simulink model "PMSM_DRIVES_SIMULATION1"  (Simulink 7.8)
settings: Solver=ode23tb  StartTime=0  StopTime=0.1  RelTol=1e-3
libraries: powerlib x6, simulink x2
settings Model: Creator=Nima  LastModifiedBy=Nima  ExtModeTrigMode=oneshot  ExtModeArmWhenConnect=off
settings DataIOCC: LimitDataPoints=off
settings OptimizationCC: BlockReduction=off  BooleanDataType=off  InitFltsAndDblsToZero=on
settings DebuggingCC: SaveWithParameterizedLinksMsg=none  SignalResolutionControl=TryResolveAllWithWarning  SolverPrmCheckMsg=none  MultiTaskDSMMsg=warning  MultiTaskCondExecSysMsg=none  FcnCallInpInsideContextMsg=Use local settings  StrictBusMsg=None
settings HardwareCC: TargetUnknown=on
settings RTWCC: IncludeERTFirstTime=on
settings GRTTargetCC: TargetFcnLib=ansi_tfl_tmw.mat

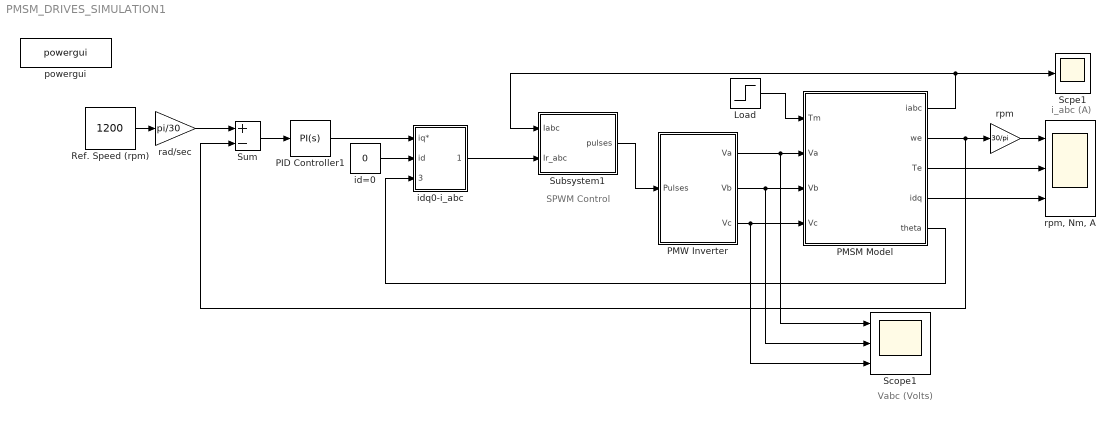
== system PMSM_DRIVES_SIMULATION1 ==
  note: i_abc (A)
  note: SPWM Control
  note: Vabc (Volts)
  " rpm" : Gain  Gain=30/pi  mask{@1=<empty>}
      mask prompts: @1 "Mask Parameter 1:"
      mask StyleString: popup(<empty>)
  Load : Step  Time=0  After=3  SampleTime=0
  PID Controller1 : simulink/Continuous/PID Controller  Controller=PI  TimeDomain=Continuous-time  SampleTime=1  IntegratorMethod=Forward Euler  FilterMethod=Forward Euler  Form=Parallel  P=10  I=2  D=0  N=100  InitialConditionSource=internal  InitialConditionForIntegrator=0  InitialConditionForFilter=0  ExternalReset=none  LimitOutput=off  UpperSaturationLimit=inf  LowerSaturationLimit=-inf  LinearizeAsGain=off  AntiWindupMode=none  Kb=1  TrackingMode=off  Kt=1  PParamMin=[]  PParamMax=[]  IParamMin=[]  IParamMax=[]  DParamMin=[]  DParamMax=[]  NParamMin=[]  NParamMax=[]  KbParamMin=[]  KbParamMax=[]  KtParamMin=[]  KtParamMax=[]  POutMin=[]  POutMax=[]  IOutMin=[]  IOutMax=[]  DOutMin=[]  DOutMax=[]  NOutMin=[]  NOutMax=[]  KbOutMin=[]  KbOutMax=[]  KtOutMin=[]  KtOutMax=[]  IntegratorOutMin=[]  IntegratorOutMax=[]  FilterOutMin=[]  FilterOutMax=[]  SumOutMin=[]  SumOutMax=[]  SumI1OutMin=[]  SumI1OutMax=[]  SumI2OutMin=[]  SumI2OutMax=[]  SumI3OutMin=[]  SumI3OutMax=[]  SumDOutMin=[]  SumDOutMax=[]  SaturationOutMin=[]  SaturationOutMax=[]  IntegratorContinuousStateAttributes=''  IntegratorStateMustResolveToSignalObject=off  IntegratorRTWStateStorageClass=Auto  FilterContinuousStateAttributes=''  FilterStateMustResolveToSignalObject=off  FilterRTWStateStorageClass=Auto
  PMSM Model : Subsystem  mask(PMSM Model ){R=1.4, Ld=0.0066, Lq=0.0058, Yaf=0.1546, J=0.00176, B=0.00038818, P=6}
      mask prompts: R "Stator Resistance R (ohm)"; Ld "Inductance  Ld ( H)"; Lq "Inductance  Lq  ( H)"; Yaf "Rotor Flux constant  Yaf (V/rad/s)"; J "Moment of inertia  J (kgm2)"; B "Friction Vicious gain B (Nm/ rad/s )"; P "Number of Poles P"
      mask help: PMSM drive with constant torque control id=0, at rated speed (60Hz), 30V DC bus voltage..
  PMW Inverter : Subsystem  mask(MOSFET/DIODE 3-Phase Bridge ){Vdc=30}
      mask prompts: Vdc "DC Bus Voltage ( Volts)"
  Ref. Speed (rpm) : Constant  Value=1200
  Scope1 : Scope  NumInputPorts=3
      settings: YMin=-5~-5~-5  YMax=5~5~5
  Scpe1 : Scope
      settings: TimeRange=1  YMin=-10  YMax=10  SaveName=ScopeData6
  Subsystem1 : Subsystem
  Sum : Sum  Inputs=+-  SaturateOnIntegerOverflow=on  InputSameDT=on  OutDataTypeStr=Inherit: Same as first input
  id=0 : Constant  Value=0
  idq0-i_abc : Subsystem  mask(Reference current generator){@1=<empty>}
      mask prompts: @1 "Mask Parameter 1:"
      mask StyleString: popup(<empty>)
  powergui : powerlib/powergui  Priority=2  SimulationMode=Continuous  SolverType=Tustin  SampleTime=0  frequency=60  SPID=off  DisableSnubberDevices=off  DisableRonSwitches=off  DisableVfSwitches=off  SwTol=0  Interpol=off  DisplayEquations=off  FunctionMessages=off  frequencyindice=0  Pbase=100e6  ErrMax=1e-4  Iterations=50  UnitsV=kV  UnitsW=MW  echomessages=off  HookPort=off  EnableUseOfTLC=off  x0status=blocks  RestoreLinks=warning  ResistiveCurrentMeasurement=off  Frange=logspace(0,3,50)  Ylog=off  Xlog=off  ShowGrid=off  save=off  variable=ZData  ZoomFFT=on  StartTime=0.0  cycles=1  DisplayStyle=off  fundamental=60  FreqAxis=off  MaxFrequency=1000  frequencyindicesteady=1  RmsSteady=1  display=off  Ts=0  methode=off
  rad/sec : Gain  Gain=pi/30  mask{@1=<empty>}
      mask prompts: @1 "Mask Parameter 1:"
      mask StyleString: popup(<empty>)
  "rpm, Nm, A" : Scope  NumInputPorts=3
      settings: TimeRange=0.1  YMin=1150~-5~-10  YMax=1240~12.5~10  SaveName=ScopeData3
  wires:
  Sum/1 -> PID Controller1/1
  Ref. Speed (rpm)/1 -> rad/sec/1
  id=0/1 -> idq0-i_abc/2(id)
  Load/1 -> PMSM Model/1(Tm)
  rad/sec/1 -> Sum/1
  PMSM Model/1(iabc) -> Scpe1/1, Subsystem1/1(Iabc)
  PMSM Model/2(we) -> " rpm"/1, Sum/2
  " rpm"/1 -> "rpm, Nm, A"/1
  PMSM Model/3(Te) -> "rpm, Nm, A"/2
  PMW Inverter/1(Va) -> PMSM Model/2(Va), Scope1/1
  PMW Inverter/2(Vb) -> PMSM Model/3(Vb), Scope1/2
  PMW Inverter/3(Vc) -> PMSM Model/4(Vc), Scope1/3
  Subsystem1/1(pulses) -> PMW Inverter/1(Pulses)
  idq0-i_abc/1(irabc) -> Subsystem1/2(Ir_abc)
  PMSM Model/5(theta) -> idq0-i_abc/3(theta)
  PMSM Model/4(idq) -> "rpm, Nm, A"/3
  PID Controller1/1 -> idq0-i_abc/1(iq*)

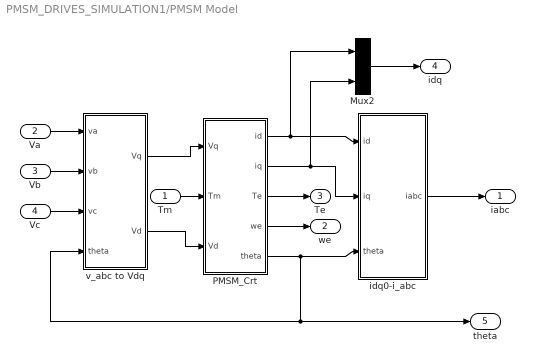
== system PMSM_DRIVES_SIMULATION1/PMSM Model ==
  Tm : Inport
  Va : Inport  Port=2
  Vb : Inport  Port=3
  Vc : Inport  Port=4
  Mux2 : Mux  Inputs=2
  PMSM_Crt : Subsystem  mask{@1=<empty>}
      mask prompts: @1 "Mask Parameter 1:"
      mask StyleString: popup(<empty>)
  idq0-i_abc : Subsystem  mask{@1=<empty>}
      mask prompts: @1 "Mask Parameter 1:"
      mask StyleString: popup(<empty>)
  v_abc to Vdq : Subsystem  mask{@1=<empty>}
      mask prompts: @1 "Mask Parameter 1:"
      mask StyleString: popup(<empty>)
  iabc : Outport
  we : Outport  Port=2
  Te : Outport  Port=3
  idq : Outport  Port=4
  theta : Outport  Port=5
  wires:
  Va/1 -> v_abc to Vdq/1(va)
  Vc/1 -> v_abc to Vdq/3(vc)
  Vb/1 -> v_abc to Vdq/2(vb)
  idq0-i_abc/1(iabc) -> iabc/1
  v_abc to Vdq/1(Vq) -> PMSM_Crt/1(Vq)
  v_abc to Vdq/2(Vd) -> PMSM_Crt/3(Vd)
  PMSM_Crt/1(id) -> idq0-i_abc/1(id), Mux2/1
  PMSM_Crt/2(iq) -> idq0-i_abc/2(iq), Mux2/2
  PMSM_Crt/5(theta) -> theta/1, v_abc to Vdq/4(theta), idq0-i_abc/3(theta)
  PMSM_Crt/4(we) -> we/1
  PMSM_Crt/3(Te) -> Te/1
  Tm/1 -> PMSM_Crt/2(Tm)
  Mux2/1 -> idq/1

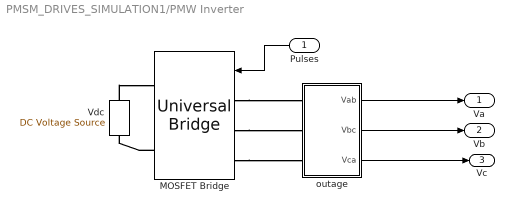
== system PMSM_DRIVES_SIMULATION1/PMW Inverter ==
  Pulses : Inport
  MOSFET Bridge : powerlib/Power Electronics/Universal Bridge  Arms=3  SnubberResistance=1e5  SnubberCapacitance=inf  Device=MOSFET / Diodes  Ron=1e-3  Lon=0  ForwardVoltages="[  0  0  ]"  ForwardVoltage=0  GTOparameters=[ 10e-6 , 20e-6 ]  IGBTparameters=[ 1e-6 , 2e-6 ]  Measurements=None  Measurements_2=None  converterType=Rectifier
  Vdc : powerlib/Electrical Sources/DC Voltage Source  Amplitude=Vdc  Measurements=None
  outage : Subsystem
  Va : Outport
  Vb : Outport  Port=2
  Vc : Outport  Port=3
  wires:
  outage/1(Vab) -> Va/1
  outage/2(Vbc) -> Vb/1
  outage/3(Vca) -> Vc/1
  Pulses/1 -> MOSFET Bridge/1
  connections:
  MOSFET Bridge/LConn1 -- outage/LConn1
  MOSFET Bridge/LConn2 -- outage/LConn2
  MOSFET Bridge/LConn3 -- outage/LConn3
  Vdc/RConn1 -- MOSFET Bridge/RConn1
  MOSFET Bridge/RConn2 -- Vdc/LConn1

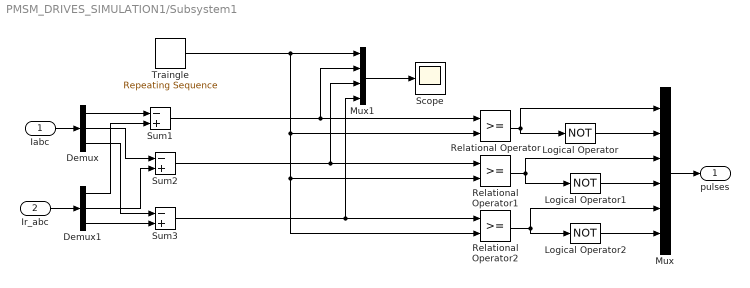
== system PMSM_DRIVES_SIMULATION1/Subsystem1 ==
  Iabc : Inport
  Ir_abc : Inport  Port=2
  Demux : Demux  Outputs=3
  Demux1 : Demux  Outputs=3
  Logical Operator : Logic  Operator=NOT
  Logical Operator1 : Logic  Operator=NOT
  Logical Operator2 : Logic  Operator=NOT
  Mux : Mux  Inputs=6
  Mux1 : Mux
  Relational Operator : RelationalOperator  OutDataTypeStr=boolean
  Relational Operator1 : RelationalOperator  OutDataTypeStr=boolean
  Relational Operator2 : RelationalOperator  OutDataTypeStr=boolean
  Scope : Scope
      settings: YMin=-100  YMax=100  SaveName=ScopeData11
  Sum1 : Sum  Inputs=-+  SaturateOnIntegerOverflow=on  InputSameDT=on  OutDataTypeStr=Inherit: Same as first input
  Sum2 : Sum  Inputs=-+  SaturateOnIntegerOverflow=on  InputSameDT=on  OutDataTypeStr=Inherit: Same as first input
  Sum3 : Sum  Inputs=-+  SaturateOnIntegerOverflow=on  InputSameDT=on  OutDataTypeStr=Inherit: Same as first input
  Traingle : simulink/Sources/Repeating Sequence  rep_seq_t=[0 1/6000/4 3/6000/4 1/6000]  rep_seq_y=[0 -30 30 0]
  pulses : Outport
  wires:
  Iabc/1 -> Demux/1
  Ir_abc/1 -> Demux1/1
  Demux/1 -> Sum1/1
  Demux1/1 -> Sum1/2
  Demux/2 -> Sum2/1
  Demux1/2 -> Sum2/2
  Demux/3 -> Sum3/1
  Demux1/3 -> Sum3/2
  Relational Operator/1 -> Logical Operator/1, Mux/1
  Logical Operator/1 -> Mux/2
  Relational Operator1/1 -> Mux/3, Logical Operator1/1
  Logical Operator1/1 -> Mux/4
  Relational Operator2/1 -> Logical Operator2/1, Mux/5
  Logical Operator2/1 -> Mux/6
  Mux/1 -> pulses/1
  Sum1/1 -> Relational Operator/1, Mux1/2
  Sum2/1 -> Relational Operator1/1, Mux1/3
  Sum3/1 -> Relational Operator2/1, Mux1/4
  Traingle/1 -> Relational Operator2/2, Relational Operator1/2, Relational Operator/2, Mux1/1
  Mux1/1 -> Scope/1

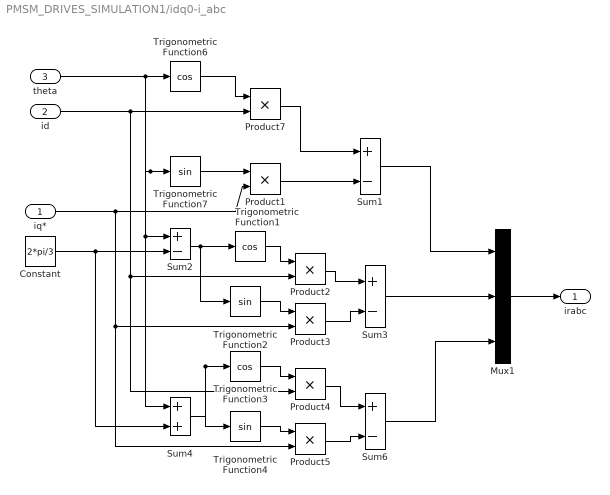
== system PMSM_DRIVES_SIMULATION1/idq0-i_abc ==
  iq* : Inport
  id : Inport  Port=2
  theta : Inport  Port=3
  Constant : Constant  Value=2*pi/3
  Mux1 : Mux  Inputs=3
  Product{1..5,7} (6 alike) : Product  SaturateOnIntegerOverflow=on  RndMeth=Zero  InputSameDT=on  OutDataTypeStr=Inherit: Same as first input
  Sum{1..3,6} (4 alike) : Sum  Inputs=+-  SaturateOnIntegerOverflow=on  InputSameDT=on  OutDataTypeStr=Inherit: Same as first input
  Sum4 : Sum  SaturateOnIntegerOverflow=on  InputSameDT=on  OutDataTypeStr=Inherit: Same as first input
  Trigonometric Function1 : Trigonometry  Operator=cos
  Trigonometric Function2 : Trigonometry
  Trigonometric Function3 : Trigonometry  Operator=cos
  Trigonometric Function4 : Trigonometry
  Trigonometric Function6 : Trigonometry  Operator=cos
  Trigonometric Function7 : Trigonometry
  irabc : Outport
  wires:
  theta/1 -> Trigonometric Function6/1, Trigonometric Function7/1, Sum2/1, Sum4/1
  Trigonometric Function6/1 -> Product7/1
  Trigonometric Function7/1 -> Product1/1
  id/1 -> Product7/2, Product2/2, Product4/2
  Product1/1 -> Sum1/2
  Product7/1 -> Sum1/1
  Sum2/1 -> Trigonometric Function1/1, Trigonometric Function2/1
  Trigonometric Function1/1 -> Product2/1
  Trigonometric Function2/1 -> Product3/1
  Product3/1 -> Sum3/2
  Product2/1 -> Sum3/1
  Sum3/1 -> Mux1/2
  Sum4/1 -> Trigonometric Function3/1, Trigonometric Function4/1
  Trigonometric Function3/1 -> Product4/1
  Trigonometric Function4/1 -> Product5/1
  Product4/1 -> Sum6/1
  Product5/1 -> Sum6/2
  Sum6/1 -> Mux1/3
  Mux1/1 -> irabc/1
  iq*/1 -> Product1/2, Product3/2, Product5/2
  Constant/1 -> Sum2/2, Sum4/2
  Sum1/1 -> Mux1/1

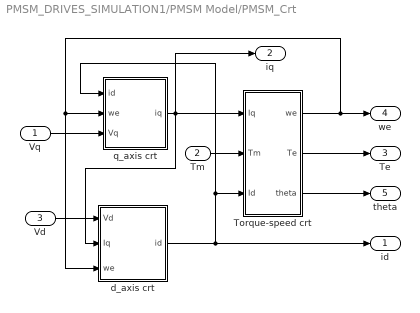
== system PMSM_DRIVES_SIMULATION1/PMSM Model/PMSM_Crt ==
  Vq : Inport
  Tm : Inport  Port=2
  Vd : Inport  Port=3
  Torque-speed crt : Subsystem  mask{@1=<empty>}
      mask prompts: @1 "Mask Parameter 1:"
      mask StyleString: popup(<empty>)
  d_axis crt : Subsystem  mask{@1=<empty>}
      mask prompts: @1 "Mask Parameter 1:"
      mask StyleString: popup(<empty>)
  q_axis crt : Subsystem  mask{@1=<empty>}
      mask prompts: @1 "Mask Parameter 1:"
      mask StyleString: popup(<empty>)
  id : Outport
  iq : Outport  Port=2
  Te : Outport  Port=3
  we : Outport  Port=4
  theta : Outport  Port=5
  wires:
  d_axis crt/1(id) -> q_axis crt/1(id), Torque-speed crt/3(Id), id/1
  Vd/1 -> d_axis crt/1(Vd)
  q_axis crt/1(iq) -> d_axis crt/2(Iq), iq/1, Torque-speed crt/1(Iq)
  Torque-speed crt/1(we) -> q_axis crt/2(we), d_axis crt/3(we), we/1
  Vq/1 -> q_axis crt/3(Vq)
  Tm/1 -> Torque-speed crt/2(Tm)
  Torque-speed crt/2(Te) -> Te/1
  Torque-speed crt/3("theta ") -> theta/1

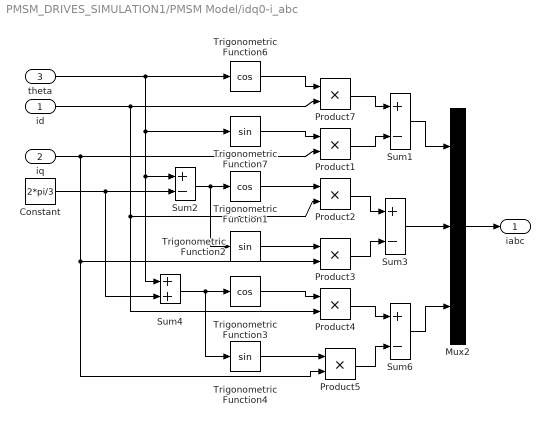
== system PMSM_DRIVES_SIMULATION1/PMSM Model/idq0-i_abc ==
  id : Inport
  iq : Inport  Port=2
  theta : Inport  Port=3
  Constant : Constant  Value=2*pi/3
  Mux2 : Mux  Inputs=3
  Product{1..5,7} (6 alike) : Product  SaturateOnIntegerOverflow=on  RndMeth=Zero  InputSameDT=on  OutDataTypeStr=Inherit: Same as first input
  Sum{1..3,6} (4 alike) : Sum  Inputs=+-  SaturateOnIntegerOverflow=on  InputSameDT=on  OutDataTypeStr=Inherit: Same as first input
  Sum4 : Sum  SaturateOnIntegerOverflow=on  InputSameDT=on  OutDataTypeStr=Inherit: Same as first input
  Trigonometric Function1 : Trigonometry  Operator=cos
  Trigonometric Function2 : Trigonometry
  Trigonometric Function3 : Trigonometry  Operator=cos
  Trigonometric Function4 : Trigonometry
  Trigonometric Function6 : Trigonometry  Operator=cos
  Trigonometric Function7 : Trigonometry
  iabc : Outport
  wires:
  theta/1 -> Trigonometric Function6/1, Trigonometric Function7/1, Sum2/1, Sum4/1
  Trigonometric Function6/1 -> Product7/1
  Trigonometric Function7/1 -> Product1/1
  id/1 -> Product7/2, Product2/2, Product4/2
  Product1/1 -> Sum1/2
  Product7/1 -> Sum1/1
  Sum2/1 -> Trigonometric Function1/1, Trigonometric Function2/1
  Trigonometric Function1/1 -> Product2/1
  Trigonometric Function2/1 -> Product3/1
  Product3/1 -> Sum3/2
  Product2/1 -> Sum3/1
  Sum4/1 -> Trigonometric Function3/1, Trigonometric Function4/1
  Trigonometric Function3/1 -> Product4/1
  Trigonometric Function4/1 -> Product5/1
  Product4/1 -> Sum6/1
  Product5/1 -> Sum6/2
  iq/1 -> Product1/2, Product3/2, Product5/2
  Constant/1 -> Sum2/2, Sum4/2
  Sum3/1 -> Mux2/2
  Sum1/1 -> Mux2/1
  Sum6/1 -> Mux2/3
  Mux2/1 -> iabc/1

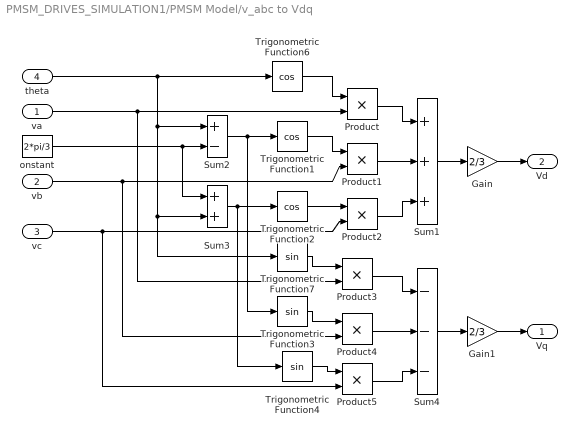
== system PMSM_DRIVES_SIMULATION1/PMSM Model/v_abc to Vdq ==
  va : Inport
  vb : Inport  Port=2
  vc : Inport  Port=3
  theta : Inport  Port=4
  Gain : Gain  Gain=2/3
  Gain1 : Gain  Gain=2/3
  Product{,1..5} (6 alike) : Product  RndMeth=Zero
  Sum1 : Sum  Inputs=+++  SaturateOnIntegerOverflow=on  InputSameDT=on  OutDataTypeStr=Inherit: Same as first input
  Sum2 : Sum  Inputs=+-  SaturateOnIntegerOverflow=on  InputSameDT=on  OutDataTypeStr=Inherit: Same as first input
  Sum3 : Sum  SaturateOnIntegerOverflow=on  InputSameDT=on  OutDataTypeStr=Inherit: Same as first input
  Sum4 : Sum  Inputs=---  SaturateOnIntegerOverflow=on  InputSameDT=on  OutDataTypeStr=Inherit: Same as first input
  Trigonometric Function1 : Trigonometry  Operator=cos
  Trigonometric Function2 : Trigonometry  Operator=cos
  Trigonometric Function3 : Trigonometry
  Trigonometric Function4 : Trigonometry
  Trigonometric Function6 : Trigonometry  Operator=cos
  Trigonometric Function7 : Trigonometry
  onstant : Constant  Value=2*pi/3
  Vq : Outport
  Vd : Outport  Port=2
  wires:
  theta/1 -> Trigonometric Function6/1, Sum2/1, Trigonometric Function7/1, Sum3/2
  Trigonometric Function6/1 -> Product/1
  va/1 -> Product/2, Product3/2
  Product/1 -> Sum1/1
  onstant/1 -> Sum2/2, Sum3/1
  Sum2/1 -> Trigonometric Function1/1, Trigonometric Function3/1
  Trigonometric Function1/1 -> Product1/1
  vb/1 -> Product1/2, Product4/2
  Product1/1 -> Sum1/2
  Sum3/1 -> Trigonometric Function2/1, Trigonometric Function4/1
  Trigonometric Function2/1 -> Product2/1
  vc/1 -> Product2/2, Product5/2
  Product2/1 -> Sum1/3
  Sum1/1 -> Gain/1
  Gain/1 -> Vd/1
  Trigonometric Function7/1 -> Product3/1
  Product3/1 -> Sum4/1
  Trigonometric Function3/1 -> Product4/1
  Product4/1 -> Sum4/2
  Trigonometric Function4/1 -> Product5/1
  Product5/1 -> Sum4/3
  Sum4/1 -> Gain1/1
  Gain1/1 -> Vq/1

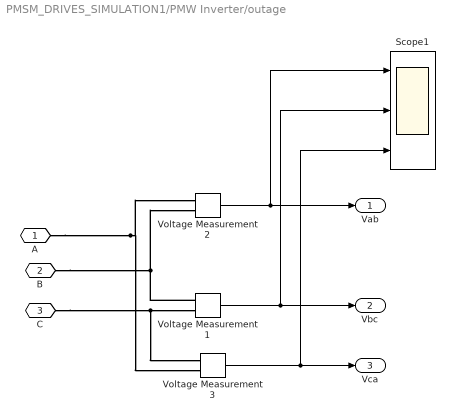
== system PMSM_DRIVES_SIMULATION1/PMW Inverter/outage ==
  Scope1 : Scope  NumInputPorts=3
      settings: YMin=-5~-5~-5  YMax=5~5~5
  Voltage Measurement1 : powerlib/Measurements/Voltage Measurement  PhasorSimulation=off  OutputType=Complex  PSBequivalent=0
  Voltage Measurement2 : powerlib/Measurements/Voltage Measurement  PhasorSimulation=off  OutputType=Complex  PSBequivalent=0
  Voltage Measurement3 : powerlib/Measurements/Voltage Measurement  PhasorSimulation=off  OutputType=Complex  PSBequivalent=0
  A : PMIOPort  Port=1  Side=Left
  B : PMIOPort  Port=2  Side=Left
  C : PMIOPort  Port=3  Side=Left
  Vab : Outport
  Vbc : Outport  Port=2
  Vca : Outport  Port=3
  wires:
  Voltage Measurement2/1 -> Vab/1, Scope1/1
  Voltage Measurement1/1 -> Vbc/1, Scope1/2
  Voltage Measurement3/1 -> Vca/1, Scope1/3
  connections:
  Voltage Measurement1/LConn1 -- Voltage Measurement2/LConn2 -- B/RConn1
  A/RConn1 -- Voltage Measurement2/LConn1 -- Voltage Measurement3/LConn2
  C/RConn1 -- Voltage Measurement1/LConn2 -- Voltage Measurement3/LConn1

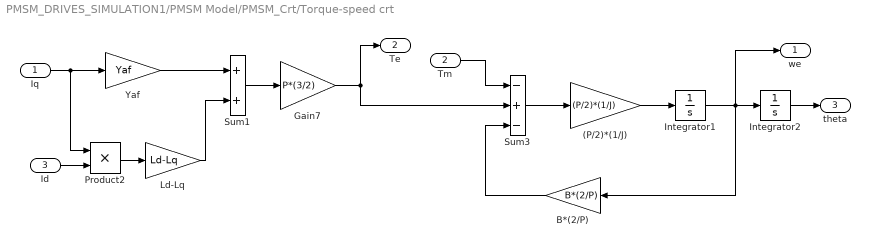
== system PMSM_DRIVES_SIMULATION1/PMSM Model/PMSM_Crt/Torque-speed crt ==
  Iq : Inport
  Tm : Inport  Port=2
  Id : Inport  Port=3
  (P/2)*(1/J) : Gain  Gain=(P/2)*(1/J)
  B*(2/P) : Gain  Gain=B*(2/P)
  Gain7 : Gain  Gain=P*(3/2)
  Integrator1 : Integrator
  Integrator2 : Integrator
  Ld-Lq : Gain  Gain=Ld-Lq
  Product2 : Product  RndMeth=Zero
  Sum1 : Sum
  Sum3 : Sum  Inputs=-+-
  Yaf : Gain  Gain=Yaf
  we : Outport
  Te : Outport  Port=2
  "theta " : Outport  Port=3
  wires:
  Yaf/1 -> Sum1/1
  Sum1/1 -> Gain7/1
  Ld-Lq/1 -> Sum1/2
  Product2/1 -> Ld-Lq/1
  Sum3/1 -> (P/2)*(1/J)/1
  Iq/1 -> Product2/1, Yaf/1
  Id/1 -> Product2/2
  Integrator1/1 -> B*(2/P)/1, Integrator2/1, we/1
  Gain7/1 -> Sum3/2, Te/1
  Tm/1 -> Sum3/1
  B*(2/P)/1 -> Sum3/3
  (P/2)*(1/J)/1 -> Integrator1/1
  Integrator2/1 -> "theta "/1

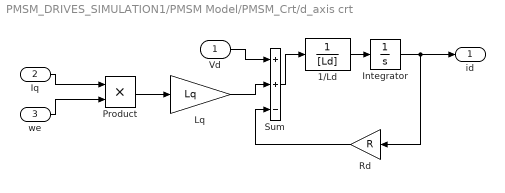
== system PMSM_DRIVES_SIMULATION1/PMSM Model/PMSM_Crt/d_axis crt ==
  Vd : Inport
  Iq : Inport  Port=2
  we : Inport  Port=3
  1/Ld : TransferFcn  Denominator=[Ld]
  Integrator : Integrator
  Lq : Gain  Gain=Lq
  Product : Product  RndMeth=Zero
  Rd : Gain  Gain=R
  Sum : Sum  Inputs=++-
  id : Outport
  wires:
  Sum/1 -> 1/Ld/1
  1/Ld/1 -> Integrator/1
  Product/1 -> Lq/1
  Iq/1 -> Product/1
  we/1 -> Product/2
  Lq/1 -> Sum/2
  Integrator/1 -> id/1, Rd/1
  Rd/1 -> Sum/3
  Vd/1 -> Sum/1

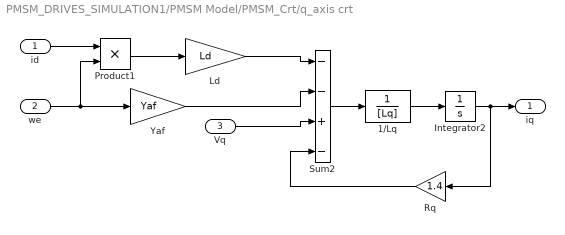
== system PMSM_DRIVES_SIMULATION1/PMSM Model/PMSM_Crt/q_axis crt ==
  id : Inport
  we : Inport  Port=2
  Vq : Inport  Port=3
  1/Lq : TransferFcn  Denominator=[Lq]
  Integrator2 : Integrator
  Ld : Gain  Gain=Ld
  Product1 : Product  RndMeth=Zero
  Rq : Gain  Gain=1.4
  Sum2 : Sum  Inputs=--+-
  Yaf : Gain  Gain=Yaf
  iq : Outport
  wires:
  Product1/1 -> Ld/1
  Vq/1 -> Sum2/3
  Sum2/1 -> 1/Lq/1
  1/Lq/1 -> Integrator2/1
  Integrator2/1 -> iq/1, Rq/1
  Rq/1 -> Sum2/4
  Ld/1 -> Sum2/1
  Yaf/1 -> Sum2/2
  we/1 -> Yaf/1, Product1/2
  id/1 -> Product1/1
